simulink model "sfcndemo_sw"  (Simulink 7.6)
settings: Solver=FixedStepDiscrete  StartTime=0.0  StopTime=4  FixedStep=1  RelTol=1e-3
Description:
  | Switch implemented in C-MEX S-function
settings Model: Creator=The MathWorks Inc.  ExtModeAutoUpdateStatusClock=off  BufferReuse=off
settings OptimizationCC: BooleanDataType=off  OptimizeBlockIOStorage=off  BufferReuse=off  ExpressionFolding=off  LocalBlockOutputs=off  InitFltsAndDblsToZero=on
settings DebuggingCC: SaveWithParameterizedLinksMsg=none  SignalResolutionControl=TryResolveAllWithWarning  SolverPrmCheckMsg=none  MultiTaskDSMMsg=warning  MultiTaskCondExecSysMsg=none
settings HardwareCC: TargetUnknown=on
settings RTWCC: IncludeERTFirstTime=on
settings CodeAppCC: CustomSymbolStrFcn=$F$N$M
settings GRTTargetCC: TargetFcnLib=ansi_tfl_tmw.mat

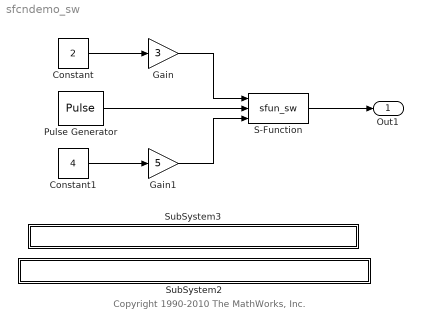
== system sfcndemo_sw ==
  note: Copyright 1990-2010 The MathWorks, Inc.
  Constant : Constant  Value=2
  Constant1 : Constant  Value=4
  Gain : Gain  Gain=3  SaturateOnIntegerOverflow=on  OutDataTypeStr=Inherit: Same as input  ParamDataTypeStr=Inherit: Same as input
  Gain1 : Gain  Gain=5  SaturateOnIntegerOverflow=on  OutDataTypeStr=Inherit: Same as input  ParamDataTypeStr=Inherit: Same as input
  Pulse Generator : DiscretePulseGenerator
  S-Function : S-Function  FunctionName=sfun_sw  EnableBusSupport=off
  SubSystem2 : Subsystem  mask{filename=sfun_sw.tlc}
      mask init:
      | x=sfundemo_maskdisp;
      settings: AttributesFormatString=\n  OpenFcn=sfundemo_openfcn
      mask Display: disp(x);
  SubSystem3 : Subsystem  mask{filename=sfun_sw.c}
      mask init:
      | x=sfundemo_maskdisp;
      settings: AttributesFormatString=\n  OpenFcn=sfundemo_openfcn
      mask Display: disp(x);
  Out1 : Outport
  wires:
  Constant/1 -> Gain/1
  Constant1/1 -> Gain1/1
  Gain/1 -> S-Function/1
  Pulse Generator/1 -> S-Function/2
  Gain1/1 -> S-Function/3
  S-Function/1 -> Out1/1

== system sfcndemo_sw/SubSystem2 ==

== system sfcndemo_sw/SubSystem3 ==
